simulink model "RLC_Circuit"  (R2022a)
settings: Solver=VariableStepAuto  StartTime=0.0  StopTime=10.0  RelTol=1e-3
undefined symbols (not defined in the file): C, L, R
settings Model: Creator=Adam Ghatta  LastModifiedBy=Adam Ghatta

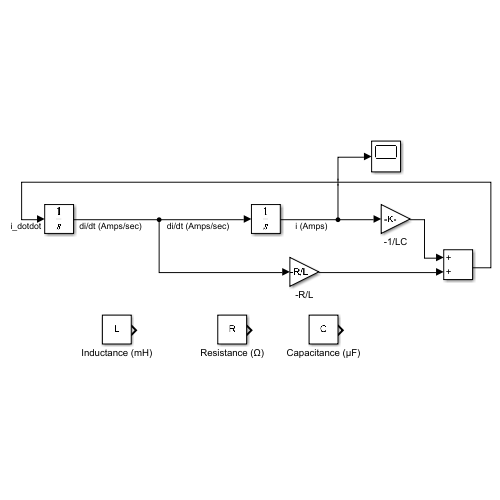
[thumbnail: Simulink's stored preview of the top-level diagram]
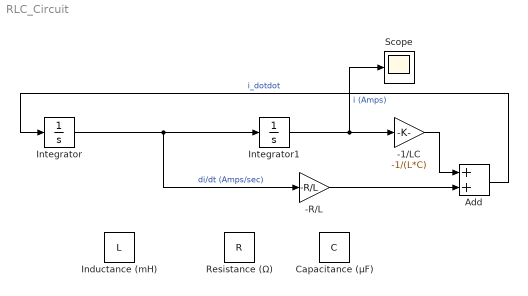
== system RLC_Circuit ==
  -1/LC : Gain  Gain=-1/(L*C)
  -R/L : Gain  Gain=-R/L
  Add : Sum
  Capacitance (μF) : Constant  Value=C
  Inductance (mH) : Constant  Value=L
  Integrator : Integrator
  Integrator1 : Integrator  InitialCondition=.1
  Resistance (Ω) : Constant  Value=R
  Scope : Scope
  wires:
  Integrator/1 -> -R/L/1, Integrator1/1  "di/dt (Amps/sec)"
  Integrator1/1 -> Scope/1, -1/LC/1  "i (Amps)"
  Add/1 -> Integrator/1  "i_dotdot"
  -1/LC/1 -> Add/1
  -R/L/1 -> Add/2
